simulink model "stateflow_s_function"  (R2018b)
settings: Solver=FixedStepDiscrete  StartTime=0.0  StopTime=10.0  FixedStep=timing.T_optiTask  RelTol=1e-3
InitFcn:
  | iiwa_joint_trajectoryfollowingcontrol_rigid_parameters;
settings Model: Creator=student  LastModifiedBy=student
settings DataIOCC: SaveOutput=off  SaveTime=off
settings OptimizationCC: DefaultParameterBehavior=Inlined

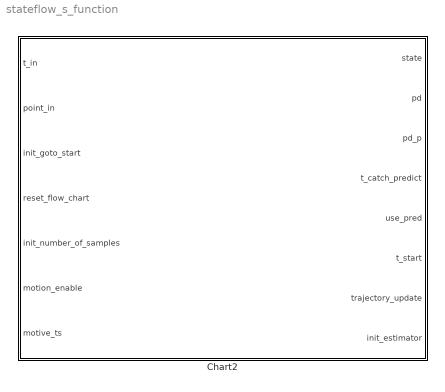
== system stateflow_s_function ==
  Chart2 : Subsystem
      mask help: Simulink:masks:GenSFuncDesc_MD
      mask Help: eval('feval(''rtwprivate'',''rtwhelpview'',''rtw_sfcn_block'')');

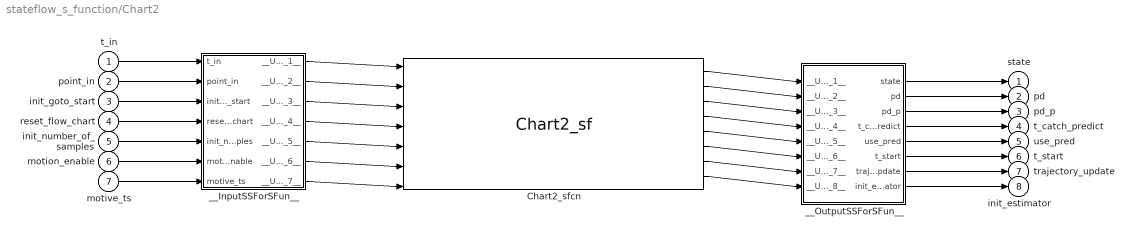
== system stateflow_s_function/Chart2 ==
  t_in : Inport
  point_in : Inport  Port=2
  init_goto_start : Inport  Port=3
  reset_flow_chart : Inport  Port=4
  init_number_of_samples : Inport  Port=5
  motion_enable : Inport  Port=6
  motive_ts : Inport  Port=7
  Chart2_sfcn : S-Function  FunctionName=Chart2_sf  SFunctionModules=""  SFunctionDeploymentMode=off  EnableBusSupport=off  mask{rtw_sf_name=Chart2_sf, showVar=off}
      mask prompts: rtw_sf_name "Simulink:masks:GenSFuncName_MP"; showVar "Simulink:masks:GenSFuncShowModuleList_MP"
      mask help: Simulink:masks:GenSFuncDesc_MD
      mask init:
      | displist = '';
      | if ~strcmp(get_param(gcb, 'FunctionName'), rtw_sf_name);
      |   set_param(gcb, 'FunctionName', rtw_sf_name);
      | end
      | % Check if we are generating code
      | rtw_mode = false;
      | if strcmpi(get_param(bdroot(gcb),'SimulationStatus'),'Initializing')
      | 	rtw_mode = strcmpi(get_param(bdroot(gcb),'BuildingRTWCode'),'on') && ...
      | 		~strcmpi(get_param(bdroot(gcb),'TargetStyle'),'SimulationTarget');
      | end
      | if showVar || rtw_mode
      | 	if exist('rtwsfunc') == 2 | exist('rtwsfunc') == 6
      | 		tmplist = rtwsfunc(rtw_sf_name,gcb);
      | 		tmplist = DAStudio.message('Simulink:masks:GenSFuncListOfModules_IC', tmplist);
      | 	elseif showVar
      | 		tmplist1 = DAStudio.message('Simulink:masks:GenSFuncListOfModules_IC', '');
      |         tmplist2 = DAStudio.message('Simulink:masks:GenSFuncNotLicensed_IC');
      |         tmplist = [tmplist1 tmplist2];
      |  	end
      | end
      | if showVar
      |   displist = tmplist;
      | end
      settings: CopyFcn=|
      | if ~strcmp(get_param(gcb,'Linkstatus'),'none') && ...
      | ~strcmp(get_param(gcb,'Linkstatus'),'implicit')
      |   set_param(gcb,'LinkStatus','none');
      | end
      mask Help: eval('feval(''rtwprivate'',''rtwhelpview'',''rtw_sfcn_block'')');
      mask Display:
      | port_label('input',1,'t_in');
      | port_label('input',2,'point_in');
      | port_label('input',3,'init_goto_start');
      | port_label('input',4,'reset_flow_chart');
      | port_label('input',5,'init_number_of_samples');
      | port_label('input',6,'motion_enable');
      | port_label('input',7,'motive_ts');
      | port_label('output',1,'state');
      | port_label('output',2,'pd');
      | port_label('output',3,'pd_p');
      | port_label('output',4,'t_catch_predict');
      | port_label('output',5,'use_pred');
      | port_label('output',6,'t_start');
      | port_label('output',7,'trajectory_update');
      | port_label('output',8,'init_estimator');
  __InputSSForSFun__ : Subsystem
  __OutputSSForSFun__ : Subsystem
  state : Outport  VectorParamsAs1DForOutWhenUnconnected=on
  pd : Outport  Port=2  VectorParamsAs1DForOutWhenUnconnected=on
  pd_p : Outport  Port=3  VectorParamsAs1DForOutWhenUnconnected=on
  t_catch_predict : Outport  Port=4  VectorParamsAs1DForOutWhenUnconnected=on
  use_pred : Outport  Port=5  VectorParamsAs1DForOutWhenUnconnected=on
  t_start : Outport  Port=6  VectorParamsAs1DForOutWhenUnconnected=on
  trajectory_update : Outport  Port=7  VectorParamsAs1DForOutWhenUnconnected=on
  init_estimator : Outport  Port=8
  wires:
  t_in/1 -> __InputSSForSFun__/1(t_in)
  point_in/1 -> __InputSSForSFun__/2(point_in)
  init_goto_start/1 -> __InputSSForSFun__/3(init_goto_start)
  reset_flow_chart/1 -> __InputSSForSFun__/4(reset_flow_chart)
  init_number_of_samples/1 -> __InputSSForSFun__/5(init_number_of_samples)
  motion_enable/1 -> __InputSSForSFun__/6(motion_enable)
  motive_ts/1 -> __InputSSForSFun__/7(motive_ts)
  __InputSSForSFun__/1(__UniqueOutportName__1__) -> Chart2_sfcn/1
  __InputSSForSFun__/2(__UniqueOutportName__2__) -> Chart2_sfcn/2
  __InputSSForSFun__/3(__UniqueOutportName__3__) -> Chart2_sfcn/3
  __InputSSForSFun__/4(__UniqueOutportName__4__) -> Chart2_sfcn/4
  __InputSSForSFun__/5(__UniqueOutportName__5__) -> Chart2_sfcn/5
  __InputSSForSFun__/6(__UniqueOutportName__6__) -> Chart2_sfcn/6
  __InputSSForSFun__/7(__UniqueOutportName__7__) -> Chart2_sfcn/7
  Chart2_sfcn/1 -> __OutputSSForSFun__/1(__UniqueInportName__1__)
  Chart2_sfcn/2 -> __OutputSSForSFun__/2(__UniqueInportName__2__)
  Chart2_sfcn/3 -> __OutputSSForSFun__/3(__UniqueInportName__3__)
  Chart2_sfcn/4 -> __OutputSSForSFun__/4(__UniqueInportName__4__)
  Chart2_sfcn/5 -> __OutputSSForSFun__/5(__UniqueInportName__5__)
  Chart2_sfcn/6 -> __OutputSSForSFun__/6(__UniqueInportName__6__)
  Chart2_sfcn/7 -> __OutputSSForSFun__/7(__UniqueInportName__7__)
  Chart2_sfcn/8 -> __OutputSSForSFun__/8(__UniqueInportName__8__)
  __OutputSSForSFun__/1(state) -> state/1
  __OutputSSForSFun__/2(pd) -> pd/1
  __OutputSSForSFun__/3(pd_p) -> pd_p/1
  __OutputSSForSFun__/4(t_catch_predict) -> t_catch_predict/1
  __OutputSSForSFun__/5(use_pred) -> use_pred/1
  __OutputSSForSFun__/6(t_start) -> t_start/1
  __OutputSSForSFun__/7(trajectory_update) -> trajectory_update/1
  __OutputSSForSFun__/8(init_estimator) -> init_estimator/1

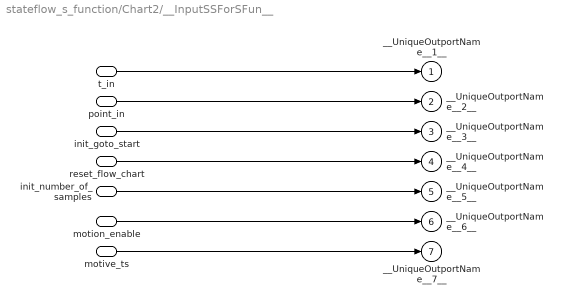
== system stateflow_s_function/Chart2/__InputSSForSFun__ ==
  t_in : Inport
  point_in : Inport  Port=2
  init_goto_start : Inport  Port=3
  reset_flow_chart : Inport  Port=4
  init_number_of_samples : Inport  Port=5
  motion_enable : Inport  Port=6
  motive_ts : Inport  Port=7
  __UniqueOutportName__1__ : Outport
  __UniqueOutportName__2__ : Outport  Port=2
  __UniqueOutportName__3__ : Outport  Port=3
  __UniqueOutportName__4__ : Outport  Port=4
  __UniqueOutportName__5__ : Outport  Port=5
  __UniqueOutportName__6__ : Outport  Port=6
  __UniqueOutportName__7__ : Outport  Port=7
  wires:
  t_in/1 -> __UniqueOutportName__1__/1
  point_in/1 -> __UniqueOutportName__2__/1
  init_goto_start/1 -> __UniqueOutportName__3__/1
  reset_flow_chart/1 -> __UniqueOutportName__4__/1
  init_number_of_samples/1 -> __UniqueOutportName__5__/1
  motion_enable/1 -> __UniqueOutportName__6__/1
  motive_ts/1 -> __UniqueOutportName__7__/1

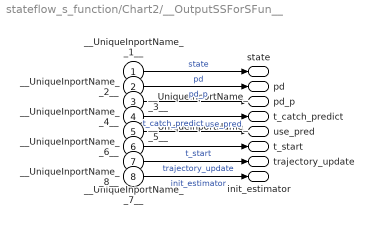
== system stateflow_s_function/Chart2/__OutputSSForSFun__ ==
  __UniqueInportName__1__ : Inport
  __UniqueInportName__2__ : Inport  Port=2
  __UniqueInportName__3__ : Inport  Port=3
  __UniqueInportName__4__ : Inport  Port=4
  __UniqueInportName__5__ : Inport  Port=5
  __UniqueInportName__6__ : Inport  Port=6
  __UniqueInportName__7__ : Inport  Port=7
  __UniqueInportName__8__ : Inport  Port=8
  state : Outport  VectorParamsAs1DForOutWhenUnconnected=on
  pd : Outport  Port=2  VectorParamsAs1DForOutWhenUnconnected=on
  pd_p : Outport  Port=3  VectorParamsAs1DForOutWhenUnconnected=on
  t_catch_predict : Outport  Port=4  VectorParamsAs1DForOutWhenUnconnected=on
  use_pred : Outport  Port=5  VectorParamsAs1DForOutWhenUnconnected=on
  t_start : Outport  Port=6  VectorParamsAs1DForOutWhenUnconnected=on
  trajectory_update : Outport  Port=7  VectorParamsAs1DForOutWhenUnconnected=on
  init_estimator : Outport  Port=8
  wires:
  __UniqueInportName__1__/1 -> state/1  "state"
  __UniqueInportName__2__/1 -> pd/1  "pd"
  __UniqueInportName__3__/1 -> pd_p/1  "pd_p"
  __UniqueInportName__4__/1 -> t_catch_predict/1  "t_catch_predict"
  __UniqueInportName__5__/1 -> use_pred/1  "use_pred"
  __UniqueInportName__6__/1 -> t_start/1  "t_start"
  __UniqueInportName__7__/1 -> trajectory_update/1  "trajectory_update"
  __UniqueInportName__8__/1 -> init_estimator/1  "init_estimator"
